simulink model "FullAdder_Block"  (R2024a)
settings: Solver=ode45  StartTime=0.0  StopTime=inf  RelTol=1e-3  EnableMultiTasking=on
settings Model: Creator=nunkesser  LastModifiedBy=nunkesser
settings SolverCC: AlgebraicLoopSolver=TrustRegion
settings DataIOCC: LimitDataPoints=on  SaveFormat=Array  ReturnWorkspaceOutputs=off
settings OptimizationCC: LifeSpan=inf
settings DebuggingCC: SolverPrmCheckMsg=warning  UnconnectedInputMsg=warning  UnconnectedOutputMsg=warning  UnconnectedLineMsg=warning  SFUnexpectedBacktrackingDiag=warning  SFNoUnconditionalDefaultTransitionDiag=warning  SFExecutionAtInitializationDiag=none  ArithmeticOperatorsInVariantConditions=warning
settings HardwareCC: ProdBitPerPointer=32  ProdBitPerSizeT=32  ProdBitPerPtrDiffT=32  ProdLargestAtomicFloat=None  ProdIntDivRoundTo=Undefined  ProdEndianess=Unspecified  ProdWordSize=32  ProdHWDeviceType=32-bit Generic
settings ModelReferenceCC: PropagateSignalLabelsOutOfModel=off
settings SFSimCC: SimUseLocalCustomCode=off  CustomCodeUndefinedFunction=UseInterfaceOnly
settings RTWCC: RTWUseLocalCustomCode=off  GPUComputeCapability=3.5
settings CodeAppCC: StateflowObjectComments=on
settings GRTTargetCC: TargetLangStandard=C89/C90 (ANSI)
settings ConfigComp: CovMetricSettings=dw  CovSaveCumulativeToWorkspaceVar=on  CovSaveSingleToWorkspaceVar=on  CovExternalEMLEnable=off  CovSFcnEnable=off

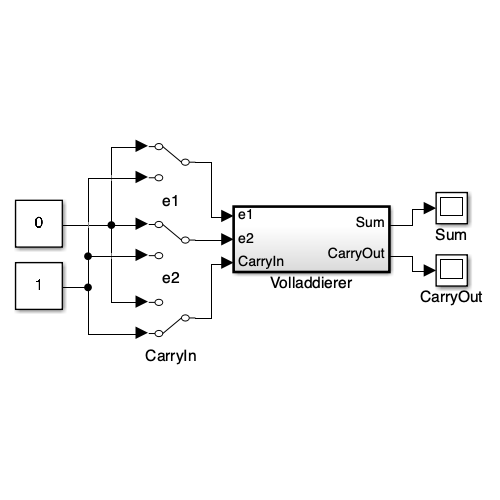
[thumbnail: Simulink's stored preview of the top-level diagram]
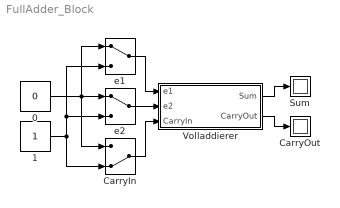
== system FullAdder_Block ==
  0 : Constant  Value=0  OutDataTypeStr=boolean
  1 : Constant  OutDataTypeStr=boolean
  CarryIn : ManualSwitch  CurrentSetting=0
  CarryOut : Display
  Sum : Display
  Volladdierer : Subsystem  TreatAsAtomicUnit=on
  e1 : ManualSwitch
  e2 : ManualSwitch
  wires:
  0/1 -> e1/1, CarryIn/1, e2/1
  1/1 -> CarryIn/2, e2/2, e1/2
  e1/1 -> Volladdierer/1(e1)
  e2/1 -> Volladdierer/2(e2)
  CarryIn/1 -> Volladdierer/3(CarryIn)
  Volladdierer/1(Sum) -> Sum/1
  Volladdierer/2(CarryOut) -> CarryOut/1

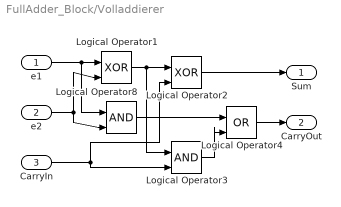
== system FullAdder_Block/Volladdierer ==
  e1 : Inport
  e2 : Inport  Port=2
  CarryIn : Inport  Port=3
  Logical Operator1 : Logic  Operator=XOR  IconShape=distinctive  AllPortsSameDT=off  OutDataTypeStr=boolean
  Logical Operator2 : Logic  Operator=XOR  IconShape=distinctive  AllPortsSameDT=off  OutDataTypeStr=boolean
  Logical Operator3 : Logic  IconShape=distinctive  AllPortsSameDT=off  OutDataTypeStr=boolean
  Logical Operator4 : Logic  Operator=OR  IconShape=distinctive  AllPortsSameDT=off  OutDataTypeStr=boolean
  Logical Operator8 : Logic  IconShape=distinctive  AllPortsSameDT=off  OutDataTypeStr=boolean
  Sum : Outport
  CarryOut : Outport  Port=2
  wires:
  e2/1 -> Logical Operator8/2, Logical Operator1/2
  Logical Operator1/1 -> Logical Operator2/1, Logical Operator3/1
  CarryIn/1 -> Logical Operator2/2, Logical Operator3/2
  Logical Operator2/1 -> Sum/1
  Logical Operator8/1 -> Logical Operator4/1
  Logical Operator3/1 -> Logical Operator4/2
  Logical Operator4/1 -> CarryOut/1
  e1/1 -> Logical Operator8/1, Logical Operator1/1
